simulink model "Motionreed"  (Simulink 7.3)
settings: Solver=ode5  StartTime=0.0  StopTime=0.5  FixedStep=Te  RelTol=1e-3
values from neighbouring files (symbols this model uses):
  c = 2*tau_amor*sqrt(k*mr)    [Paramètres_problème.m]    (also in accomodel.m = 4.685)
  c0 = 340    [Paramètres_problème.m]
  e0 = 1e-4    (= 0.0001)    [Paramètres_problème.m]
  h = 25e-4    (= 0.0025)    [Paramètres_problème.m]    (also in accomodel.m = h^N)
  k = ((2*pi*f)^2)*mr    [Paramètres_problème.m]    (also in accomodel.m = 0)
  l = 280e-4    (= 0.028)    [Paramètres_problème.m]
  mf = (8/(9*pi))*rho_0*l*h*(l^2+l*h+h^2)/(l+h)    (= 4.15595781194e-07)    [Paramètres_problème.m]
  mr = 11.4e-6    (= 1.14e-05)    [Paramètres_problème.m]
  P0 = 40    [Paramètres_problème.m]
  R = (sqrt(1./((f1.^2-f_cav^2).^2+bt.*f1.^2)))'    [Paramètres_problème.m]
  rho_0 = 1.2    [Paramètres_problème.m]
  x1 = 20e-4    (= 0.002)    [Paramètres_problème.m]
  xb = 180    [Paramètres_problème.m]
  y0 = 2e-4    (= 0.0002)    [Paramètres_problème.m]
settings Model: Creator=maison  LastModifiedBy=maison
settings DataIOCC: MaxDataPoints=100000

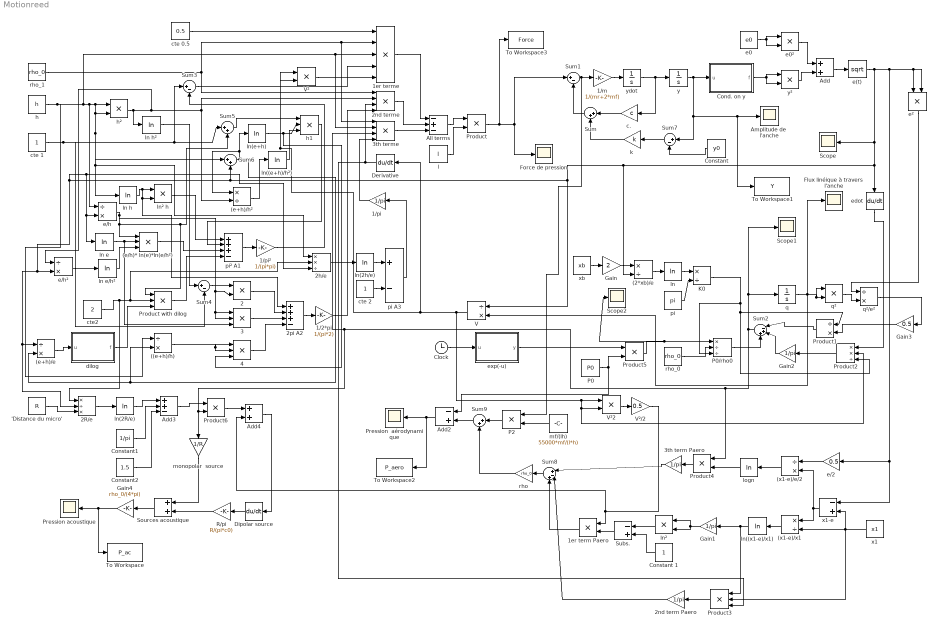
== system Motionreed ==
  'Distance du micro' : Constant  Value=R  OutDataType=fixdt(1, 16)  OutScaling=2^0
  ((e+h)/h) : Product  Inputs=/*  OutDataType=fixdt(1, 16)  OutScaling=2^-10
  (2*xb)/e : Product  Inputs=*/  OutDataType=fixdt(1, 16)  OutScaling=2^-10
  (e+h)/e : Product  Inputs=/*  OutDataType=fixdt(1, 16)  OutScaling=2^-10
  (e+h)/h² : Product  Inputs=*/  OutDataType=fixdt(1, 16)  OutScaling=2^-10
  (e/h)* ln(e)*ln(e/h²) : Product  Inputs=3  OutDataType=fixdt(1, 16)  OutScaling=2^0  RndMeth=Zero
  (x1-e)/e/2 : Product  Inputs=/*  OutDataType=fixdt(1, 16)  OutScaling=2^0  RndMeth=Zero
  (x1-e)/x1 : Product  Inputs=*/  OutDataType=fixdt(1, 16)  OutScaling=2^-10
  1/2*pi : Gain  Gain=1/(pi*2)  ParameterDataType=fixdt(1, 16)  ParameterScaling=2^0  OutDataType=fixdt(1, 16)  OutScaling=2^0
  1/m : Gain  Gain=1/(mr+2*mf)  ParameterDataType=fixdt(1, 16)  ParameterScaling=2^0  OutDataType=fixdt(1, 16)  OutScaling=2^0
  1/pi : Gain  Gain=1/pi  ParameterDataType=fixdt(1, 16)  ParameterScaling=2^0  OutDataType=fixdt(1, 16)  OutScaling=2^0
  1/pi² : Gain  Gain=1/(pi*pi)  ParameterDataType=fixdt(1, 16)  ParameterScaling=2^0  OutDataType=fixdt(1, 16)  OutScaling=2^0
  1er term Paero : Product  OutDataType=fixdt(1, 16)  OutScaling=2^0  RndMeth=Zero
  1er terme : Product  Inputs=5  OutDataType=fixdt(1, 16)  OutScaling=2^0  RndMeth=Zero
  2 : Product  OutDataType=fixdt(1, 16)  OutScaling=2^0  RndMeth=Zero
  2R/e : Product  Inputs=*/*  OutDataType=fixdt(1, 16)  OutScaling=2^0  RndMeth=Zero
  2h/e : Product  Inputs=**/  OutDataType=fixdt(1, 16)  OutScaling=2^0  RndMeth=Zero
  2nd term Paero : Gain  Gain=1/pi  ParameterDataType=fixdt(1, 16)  ParameterScaling=2^0  OutDataType=fixdt(1, 16)  OutScaling=2^0
  2nd terme : Product  Inputs=4  OutDataType=fixdt(1, 16)  OutScaling=2^0  RndMeth=Zero
  2pi A2 : Sum  Inputs=+++-  OutDataType=fixdt(1, 16)  OutScaling=2^-10
  3 : Product  Inputs=3  OutDataType=fixdt(1, 16)  OutScaling=2^0  RndMeth=Zero
  3th term Paero : Gain  Gain=1/pi  ParameterDataType=fixdt(1, 16)  ParameterScaling=2^0  OutDataType=fixdt(1, 16)  OutScaling=2^0
  3th terme : Product  Inputs=4  OutDataType=fixdt(1, 16)  OutScaling=2^0  RndMeth=Zero
  4 : Product  Inputs=3  OutDataType=fixdt(1, 16)  OutScaling=2^0  RndMeth=Zero
  Add : Sum  OutDataType=fixdt(1, 16)  OutScaling=2^-10
  Add2 : Sum  Inputs=-+  OutDataType=fixdt(1, 16)  OutScaling=2^-10
  Add3 : Sum  Inputs=++-  OutDataType=fixdt(1, 16)  OutScaling=2^-10
  Add4 : Sum  OutDataType=fixdt(1, 16)  OutScaling=2^-10
  All terms : Sum  Inputs=-+-  OutDataType=fixdt(1, 16)  OutScaling=2^-10
  Amplitude de  l'anche : Scope
      settings: YMin=-0.00125  YMax=0.0015
  Clock : Clock
      settings: Decimation=10
  Cond. on y : Stateflow chart
  Constant : Constant  Value=y0  OutDataType=fixdt(1, 16)  OutScaling=2^0
  Constant 1 : Constant  OutDataType=fixdt(1, 16)  OutScaling=2^0
  Constant1 : Constant  Value=1/pi  OutDataType=fixdt(1, 16)  OutScaling=2^0
  Constant2 : Constant  Value=1.5  OutDataType=fixdt(1, 16)  OutScaling=2^0
  Derivative : Derivative
  Dipolar source : Derivative
  Flux linéique à travers l'anche : Scope
      settings: YMin=0.0008  YMax=0.003  SaveName=ScopeData4
  Force de pression : Scope
      settings: YMin=-0.0022  YMax=-0.0003  SaveName=ScopeData2
  Gain : Gain  Gain=2  ParameterDataType=fixdt(1, 16)  ParameterScaling=2^0  OutDataType=fixdt(1, 16)  OutScaling=2^0
  Gain1 : Gain  Gain=1/pi  ParameterDataType=fixdt(1, 16)  ParameterScaling=2^0  OutDataType=fixdt(1, 16)  OutScaling=2^0
  Gain2 : Gain  Gain=1/pi  ParameterDataType=fixdt(1, 16)  ParameterScaling=2^0  OutDataType=fixdt(1, 16)  OutScaling=2^0
  Gain3 : Gain  Gain=0.5  ParameterDataType=fixdt(1, 16)  ParameterScaling=2^0  OutDataType=fixdt(1, 16)  OutScaling=2^0
  Gain4 : Gain  Gain=rho_0/(4*pi)  ParameterDataType=fixdt(1, 16)  ParameterScaling=2^0  OutDataType=fixdt(1, 16)  OutScaling=2^0
  K0 : Product  Inputs=*/  OutDataType=fixdt(1, 16)  OutScaling=2^-10
  P0 : Constant  Value=P0  OutDataType=fixdt(1, 16)  OutScaling=2^0
  P0/rho0 : Product  Inputs=*//  OutDataType=fixdt(1, 16)  OutScaling=2^-10
  P2 : Product  OutDataType=fixdt(1, 16)  OutScaling=2^0  RndMeth=Zero
  Pression acoustique : Scope
      settings: SaveName=ScopeData6
  "Pression  aérodynamique " : Scope
      settings: YMin=-25  YMax=50
  Product{,4..6} (4 alike) : Product  OutDataType=fixdt(1, 16)  OutScaling=2^0  RndMeth=Zero
  Product with dilog : Product  Inputs=3  OutDataType=fixdt(1, 16)  OutScaling=2^0  RndMeth=Zero
  Product1 : Product  Inputs=/*  OutDataType=fixdt(1, 16)  OutScaling=2^0  RndMeth=Zero
  Product2 : Product  Inputs=**/  OutDataType=fixdt(1, 16)  OutScaling=2^0  RndMeth=Zero
  Product3 : Product  Inputs=3  OutDataType=fixdt(1, 16)  OutScaling=2^0  RndMeth=Zero
  R/pi : Gain  Gain=R/(pi*c0)  ParameterDataType=fixdt(1, 16)  ParameterScaling=2^0  OutDataType=fixdt(1, 16)  OutScaling=2^0
  Scope : Scope
      settings: YMin=0.0001  YMax=0.0015  SaveName=ScopeData3
  Scope1 : Scope
      settings: SaveName=ScopeData5
  Scope2 : Scope
      settings: YMin=0  YMax=40  SaveName=ScopeData7
  Sources acoustique : Sum  OutDataType=fixdt(1, 16)  OutScaling=2^-10
  Subs. : Sum  Inputs=-+  OutDataType=fixdt(1, 16)  OutScaling=2^-10
  Sum{,5..6,9} (4 alike) : Sum  Inputs=|++  OutDataType=fixdt(1, 16)  OutScaling=2^0
  Sum{1,3..4,7} (4 alike) : Sum  Inputs=|+-  OutDataType=fixdt(1, 16)  OutScaling=2^0
  Sum2 : Sum  Inputs=|-++  OutDataType=fixdt(1, 16)  OutScaling=2^0
  Sum8 : Sum  Inputs=|+-+  OutDataType=fixdt(1, 16)  OutScaling=2^0
  To Workspace : ToWorkspace  VariableName=P_ac  SampleTime=-1  SaveFormat=Structure With Time
  To Workspace1 : ToWorkspace  VariableName=Y  SampleTime=-1  SaveFormat=Structure With Time
  To Workspace2 : ToWorkspace  VariableName=P_aero  SampleTime=-1  SaveFormat=Structure With Time
  To Workspace3 : ToWorkspace  VariableName=Force  SampleTime=-1  SaveFormat=Structure
  V : Product  Inputs=/*  OutDataType=fixdt(1, 16)  OutScaling=2^-10
  V² : Product  OutDataType=fixdt(1, 16)  OutScaling=2^0  RndMeth=Zero
  V²/2 : Gain  Gain=0.5  ParameterDataType=fixdt(1, 16)  ParameterScaling=2^0  OutDataType=fixdt(1, 16)  OutScaling=2^0
  V²2 : Product  OutDataType=fixdt(1, 16)  OutScaling=2^0  RndMeth=Zero
  c. : Gain  Gain=c  ParameterDataType=fixdt(1, 16)  ParameterScaling=2^0  OutDataType=fixdt(1, 16)  OutScaling=2^0
  cte 0.5 : Constant  Value=0.5  OutDataType=fixdt(1, 16)  OutScaling=2^0
  cte 1 : Constant  OutDataType=fixdt(1, 16)  OutScaling=2^0
  cte 2 : Constant  OutDataType=fixdt(1, 16)  OutScaling=2^0
  cte2 : Constant  Value=2  OutDataType=fixdt(1, 16)  OutScaling=2^0
  dilog : Stateflow chart
  e(t) : Math  Operator=sqrt  OutDataType=fixdt(1, 16)  OutScaling=2^0  SaturateOnIntegerOverflow=on
  e/2 : Gain  Gain=0.5  ParameterDataType=fixdt(1, 16)  ParameterScaling=2^0  OutDataType=fixdt(1, 16)  OutScaling=2^0
  e/h : Product  Inputs=/*  OutDataType=fixdt(1, 16)  OutScaling=2^-10
  e/h² : Product  Inputs=/*  OutDataType=fixdt(1, 16)  OutScaling=2^-10
  e0 : Constant  Value=e0  OutDataType=fixdt(1, 16)  OutScaling=2^0
  e0² : Product  Inputs=**  OutDataType=fixdt(1, 16)  OutScaling=2^-10
  edot : Derivative
  exp(-u) : Stateflow chart
  e² : Product  OutDataType=fixdt(1, 16)  OutScaling=2^0  RndMeth=Zero
  h : Constant  Value=h  OutDataType=fixdt(1, 16)  OutScaling=2^0
  h1 : Product  Inputs=3  OutDataType=fixdt(1, 16)  OutScaling=2^0  RndMeth=Zero
  h² : Product  OutDataType=fixdt(1, 16)  OutScaling=2^0  RndMeth=Zero
  k : Gain  Gain=k  ParameterDataType=fixdt(1, 16)  ParameterScaling=2^0  OutDataType=fixdt(1, 16)  OutScaling=2^0
  l : Constant  Value=l  OutDataType=fixdt(1, 16)  OutScaling=2^0
  ln : Math  Operator=log  OutDataType=fixdt(1, 16)  OutScaling=2^0  SaturateOnIntegerOverflow=on
  ln e : Math  Operator=log  OutDataType=fixdt(1, 16)  OutScaling=2^0  SaturateOnIntegerOverflow=on
  ln e/h² : Math  Operator=log  OutDataType=fixdt(1, 16)  OutScaling=2^0  SaturateOnIntegerOverflow=on
  ln h : Math  Operator=log  OutDataType=fixdt(1, 16)  OutScaling=2^0  SaturateOnIntegerOverflow=on
  ln h² : Math  Operator=log  OutDataType=fixdt(1, 16)  OutScaling=2^0  SaturateOnIntegerOverflow=on
  ln((e+h)/h²) : Math  Operator=log  OutDataType=fixdt(1, 16)  OutScaling=2^0  SaturateOnIntegerOverflow=on
  ln((x1-e)/x1) : Math  Operator=log  OutDataType=fixdt(1, 16)  OutScaling=2^0  SaturateOnIntegerOverflow=on
  ln(2R/e) : Math  Operator=log  OutDataType=fixdt(1, 16)  OutScaling=2^0  SaturateOnIntegerOverflow=on
  ln(2h/e) : Math  Operator=log  OutDataType=fixdt(1, 16)  OutScaling=2^0  SaturateOnIntegerOverflow=on
  ln(e+h) : Math  Operator=log  OutDataType=fixdt(1, 16)  OutScaling=2^0  SaturateOnIntegerOverflow=on
  ln² : Product  OutDataType=fixdt(1, 16)  OutScaling=2^0  RndMeth=Zero
  ln² h : Product  OutDataType=fixdt(1, 16)  OutScaling=2^0  RndMeth=Zero
  logn : Math  Operator=log  OutDataType=fixdt(1, 16)  OutScaling=2^0  SaturateOnIntegerOverflow=on
  mf/(lh) : Constant  Value=55000*mf/(l*h)  OutDataType=fixdt(1, 16)  OutScaling=2^0
  monopolar  source : Gain  Gain=1/R  ParameterDataType=fixdt(1, 16)  ParameterScaling=2^0  OutDataType=fixdt(1, 16)  OutScaling=2^0
  pi : Constant  Value=pi  OutDataType=fixdt(1, 16)  OutScaling=2^0
  pi A3 : Sum  Inputs=+-  OutDataType=fixdt(1, 16)  OutScaling=2^-10
  pi² A1 : Sum  Inputs=+++-  OutDataType=fixdt(1, 16)  OutScaling=2^-10
  q : Integrator
  q² : Product  OutDataType=fixdt(1, 16)  OutScaling=2^0  RndMeth=Zero
  q²/e² : Product  Inputs=/*  OutDataType=fixdt(1, 16)  OutScaling=2^0  RndMeth=Zero
  rho : Gain  Gain=rho_0  ParameterDataType=fixdt(1, 16)  ParameterScaling=2^0  OutDataType=fixdt(1, 16)  OutScaling=2^0
  rho_0 : Constant  Value=rho_0  OutDataType=fixdt(1, 16)  OutScaling=2^0
  rho_1 : Constant  Value=rho_0  OutDataType=fixdt(1, 16)  OutScaling=2^0
  x1 : Constant  Value=x1  OutDataType=fixdt(1, 16)  OutScaling=2^0
  x1-e : Sum  Inputs=-+  OutDataType=fixdt(1, 16)  OutScaling=2^-10
  xb : Constant  Value=xb  OutDataType=fixdt(1, 16)  OutScaling=2^0
  y : Integrator  InitialCondition=y0
  ydot : Integrator
  y² : Product  Inputs=**  OutDataType=fixdt(1, 16)  OutScaling=2^-10
  wires:
  ydot/1 -> y/1, c./1
  y/1 -> Cond. on y/1(u), Sum7/1, Amplitude de  l'anche/1, To Workspace1/1
  c./1 -> Sum/1
  k/1 -> Sum/2
  Sum/1 -> Sum1/2
  Sum1/1 -> 1/m/1, P2/1
  1/m/1 -> ydot/1
  y²/1 -> Add/2
  e0²/1 -> Add/1
  Add/1 -> e(t)/1
  xb/1 -> Gain/1
  Gain/1 -> (2*xb)/e/1
  e(t)/1 -> e/h²/2, (e+h)/e/1, 2R/e/2, e/h/2, ln e/1, 2h/e/3, Sum6/2, V/1, (2*xb)/e/2, edot/1, Scope/1, x1-e/1, e/2/1, e²/1, e²/2
  (2*xb)/e/1 -> ln/1
  ln/1 -> K0/1
  pi/1 -> K0/2
  rho_0/1 -> P0/rho0/2
  Sum2/1 -> Product4/1, 3th terme/3, Product6/2, monopolar  source/1, Scope1/1, q/1
  h/1 -> ((e+h)/h)/1, h²/1, h²/2, Sum6/1, ln h/1, 2h/e/1, e/h/1, 1er terme/3, 3th terme/2
  cte 0.5/1 -> 1er terme/1
  rho_1/1 -> 2nd terme/1, 1er terme/2, 3th terme/1
  h²/1 -> ln h²/1, e/h²/1, (e+h)/h²/2, 2nd terme/2
  cte 1/1 -> Sum3/1, Sum5/1, Sum4/2
  ln h/1 -> ln² h/1, ln² h/2, 2pi A2/1
  Sum3/1 -> 1er terme/4
  Sum5/1 -> h1/1
  Sum6/1 -> ln(e+h)/1, (e+h)/h²/1, ((e+h)/h)/2, (e+h)/e/2
  ln(e+h)/1 -> h1/2, 4/3
  ln((e+h)/h²)/1 -> h1/3
  ln² h/1 -> pi² A1/1
  (e+h)/h²/1 -> ln((e+h)/h²)/1
  h1/1 -> pi² A1/2
  e/h/1 -> (e/h)* ln(e)*ln(e/h²)/1, Sum5/2, Product with dilog/1, 2/2, 3/1, 3/2
  (e/h)* ln(e)*ln(e/h²)/1 -> pi² A1/3
  cte2/1 -> Product with dilog/2, 2h/e/2, 2R/e/1
  (e+h)/e/1 -> dilog/1(u)
  Product with dilog/1 -> pi² A1/4
  pi² A1/1 -> 1/pi²/1
  1/pi²/1 -> Sum3/2
  1er terme/1 -> All terms/1
  ln h²/1 -> Sum4/1
  Sum4/1 -> 2/1
  2/1 -> 2pi A2/2
  3/1 -> 2pi A2/3
  ((e+h)/h)/1 -> 4/1, 4/2
  4/1 -> 2pi A2/4
  2pi A2/1 -> 1/2*pi/1
  1/2*pi/1 -> 2nd terme/4
  Derivative/1 -> 2nd terme/3, Product3/3
  2nd terme/1 -> All terms/2
  pi A3/1 -> 1/pi/1
  1/pi/1 -> 3th terme/4
  2h/e/1 -> ln(2h/e)/1
  ln(2h/e)/1 -> pi A3/1
  cte 2/1 -> pi A3/2
  V²/1 -> 1er terme/5
  Product/1 -> Sum1/1, Force de pression/1, To Workspace3/1
  All terms/1 -> Product/1
  l/1 -> Product/2
  e0/1 -> e0²/1, e0²/2
  Cond. on y/1(f) -> y²/1, y²/2
  V/1 -> V²2/1, V²2/2, Product2/2, V²/1, V²/2, Derivative/1
  Constant/1 -> Sum7/2
  Sum7/1 -> k/1
  V²2/1 -> V²/2/1
  V²/2/1 -> 1er term Paero/1, Add4/2
  q/1 -> V/2, q²/1, q²/2, Flux linéique à travers l'anche/1
  P0/rho0/1 -> Sum2/3
  edot/1 -> Product2/1
  Product2/1 -> Gain2/1
  x1/1 -> x1-e/2, (x1-e)/x1/2, Product3/2
  x1-e/1 -> (x1-e)/x1/1, (x1-e)/e/2/2
  (x1-e)/x1/1 -> ln((x1-e)/x1)/1
  ln((x1-e)/x1)/1 -> Gain1/1, Product3/1
  Gain1/1 -> ln²/1, ln²/2
  ln²/1 -> Subs./1
  Constant 1/1 -> Subs./2
  Subs./1 -> 1er term Paero/2
  Product3/1 -> 2nd term Paero/1
  e/2/1 -> (x1-e)/e/2/1
  (x1-e)/e/2/1 -> logn/1
  logn/1 -> Product4/2
  Product4/1 -> 3th term Paero/1
  1er term Paero/1 -> Sum8/3
  3th term Paero/1 -> Sum8/1
  2nd term Paero/1 -> Sum8/2
  Sum8/1 -> rho/1
  rho/1 -> Sum9/2
  mf/(lh)/1 -> P2/2
  dilog/1(f) -> Product with dilog/3
  Clock/1 -> exp(-u)/1(u)
  P0/1 -> Product5/2, Add2/1
  Product5/1 -> P0/rho0/1, Scope2/1
  K0/1 -> P0/rho0/3, Product1/1, Product2/3
  e/h²/1 -> ln e/h²/1
  ln e/h²/1 -> (e/h)* ln(e)*ln(e/h²)/3
  ln e/1 -> (e/h)* ln(e)*ln(e/h²)/2, 3/3
  q²/1 -> q²/e²/2
  e²/1 -> q²/e²/1
  q²/e²/1 -> Gain3/1
  Gain3/1 -> Product1/2
  3th terme/1 -> All terms/3
  Product1/1 -> Sum2/1
  Add2/1 -> "Pression  aérodynamique "/1, To Workspace2/1
  Sum9/1 -> Add2/2
  'Distance du micro'/1 -> 2R/e/3
  2R/e/1 -> ln(2R/e)/1
  ln(2R/e)/1 -> Add3/1
  Constant1/1 -> Add3/2
  Constant2/1 -> Add3/3
  Add3/1 -> Product6/1
  Product6/1 -> Add4/1
  Add4/1 -> Dipolar source/1
  Dipolar source/1 -> R/pi/1
  monopolar  source/1 -> Sources acoustique/1
  R/pi/1 -> Sources acoustique/2
  Sources acoustique/1 -> Gain4/1
  Gain4/1 -> Pression acoustique/1, To Workspace/1
  Gain2/1 -> Sum2/2
  exp(-u)/1(y) -> Product5/1
  P2/1 -> Sum9/1

== matlab function Cond. on y ==
  data: u input double; f output double
function f = distgap(u)
if u>0 
    f=u;
else
    f=0;
end

== matlab function dilog ==
  data: u input double; f output double
function f = dilog2(u)
N=100;
h=(u-1)/N;
g=zeros(1,2*N);
g(1)=-1;
x=zeros(1,2*N);
x(1)=1;
x(2)=x(1)+h;
x(3)=x(2)+h;
i=2;
while x(i)<u
    g(i)=log(x(i+1))/(1-x(i+1))+log(x(i))/(1-x(i));
    x(i+2)=x(i+1)+h;
    i=i+1;
end

f=(h/2)*sum(g);

== matlab function exp(-u) ==
  data: u input double; y output double
function y = fcn(u)
s=100;
if u<2.85
y = 1-exp(-u*s);
else
    y=exp(-(u-2.85)*s);
end
